simulink model "E3"  (R2023a)
settings: Solver=VariableStepAuto  StartTime=0.0  StopTime=0.08  MaxStep=1e-4  RelTol=1e-3
undefined symbols (not defined in the file): alpha
libraries: spsDetailedThyristorLib x4, spsACVoltageSourceLib x1, spsMeanLib x1, spsSeriesRLCBranchLib x1, spsVoltageMeasurementLib x1, sps_lib x1
settings Model: Creator=swara  LastModifiedBy=swara

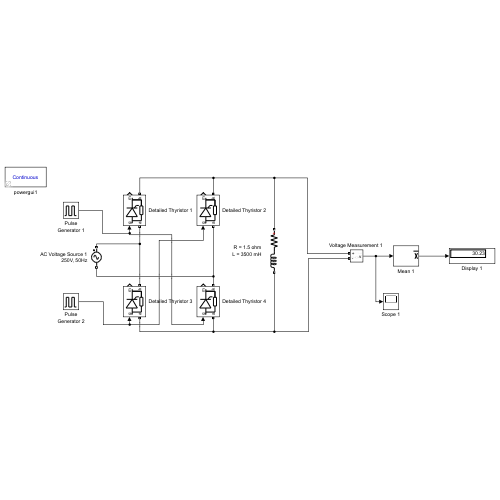
[thumbnail: Simulink's stored preview of the top-level diagram]
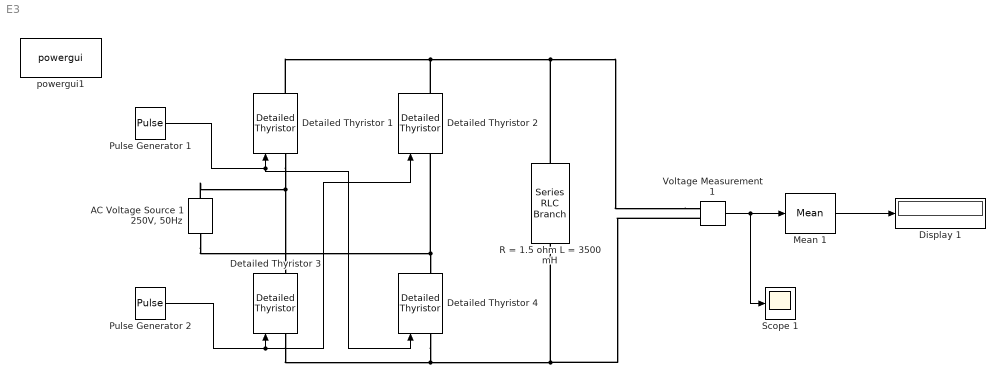
== system E3 ==
  "AC Voltage Source 1 250V, 50Hz" : spsACVoltageSourceLib/AC Voltage Source  Amplitude=100  Phase=0  Frequency=50  SampleTime=0  Measurements=None  BusType=swing  Pref=10e3  Qref=0  Qmin=-inf  Qmax=+inf
  Detailed Thyristor {1..4} (4 alike) : spsDetailedThyristorLib/Detailed Thyristor  Ron=0.001  Lon=1e-3  Vf=0.8  IL=0.1  Tq=100e-6  IC=0  Rs=500  Cs=250e-9  Measurements=on
      settings: LibrarySourceBlock=sps_lib/Power Electronics/Detailed Thyristor
  Display 1 : Display
  Mean 1 : spsMeanLib/Mean  Freq=50  Vinit=0  Ts=0
  Pulse Generator 1 : DiscretePulseGenerator  PulseType=Time based  Period=0.02  PulseWidth=5  PhaseDelay=alpha/360*0.02
  Pulse Generator 2 : DiscretePulseGenerator  PulseType=Time based  Period=0.02  PulseWidth=5  PhaseDelay=(alpha+180)/360*0.02
  R = 1.5 ohm L = 3500 mH : spsSeriesRLCBranchLib/Series RLC Branch  LConnTagsString=__new0  RConnTagsString=__new0  BranchType=RL  Resistance=1.5  Inductance=3.5  SetiL0=off  InitialCurrent=0  Capacitance=1e-6  Setx0=off  InitialVoltage=0  Measurements=None
  Scope 1 : Scope
  "Voltage Measurement 1 " : spsVoltageMeasurementLib/Voltage Measurement  PhasorSimulation=off  OutputType=Complex  PSBequivalent=0
  powergui1 : sps_lib/powergui  Priority=1  SimulationMode=Continuous  SampleTime=50e-6  frequency=60  Iterations=50  frequencyindice=50  Pbase=100e6  ErrMax=1e-4  UnitsV=kV  UnitsW=MW  buscounter=0  FunctionMessages=off  echomessages=off  EnableUseOfTLC=off  CurrentSourceSwitches=off  DisableSnubberDevices=off  DisableRonSwitches=off  DisableVfSwitches=off  DisplayEquations=off  AutomaticDiscreteSolvers=off  SolverType=Tustin/Backward Euler (TBE)  Interpol=off  ExternalGateDelay=off  methode=off  Ts=100  x0status=zero  SPID=on  SwTol=0  HookPort=off  NonlinearTolerance=1e-4  nMaxIteration=100  ContinueOnMaxIteration=off  RestoreLinks=warning  ResistiveCurrentMeasurement=off  Frange=[0:2:500]  Ylog=off  Xlog=on  ShowGrid=off  save=off  variable=ZData  structure=0  ZoomFFT=off  StartTime=0.0  cycles=1  DisplayStyle=1  fundamental=60  FreqAxis=off  MaxFrequency=1000  frequencyindicesteady=1  RmsSteady=1  display=off
  wires:
  "Voltage Measurement 1 "/1 -> Scope 1/1, Mean 1/1
  Mean 1/1 -> Display 1/1
  Pulse Generator 1/1 -> Detailed Thyristor 4/1, Detailed Thyristor 1/1
  Pulse Generator 2/1 -> Detailed Thyristor 2/1, Detailed Thyristor 3/1
  connections:
  "Voltage Measurement 1 "/LConn1 -- R = 1.5 ohm L = 3500 mH/LConn1 -- Detailed Thyristor 2/RConn1 -- Detailed Thyristor 1/RConn1
  "Voltage Measurement 1 "/LConn2 -- R = 1.5 ohm L = 3500 mH/RConn1 -- Detailed Thyristor 3/LConn1 -- Detailed Thyristor 4/LConn1
  "AC Voltage Source 1 250V, 50Hz"/LConn1 -- Detailed Thyristor 2/LConn1 -- Detailed Thyristor 4/RConn1
  "AC Voltage Source 1 250V, 50Hz"/RConn1 -- Detailed Thyristor 1/LConn1 -- Detailed Thyristor 3/RConn1
